simulink model "circuitExample"  (R2021b)
settings: Solver=VariableStepAuto  StartTime=0.0  StopTime=10.0  RelTol=1e-6
libraries: fl_lib x8, nesl_utility x1
settings Model: Creator=Rocksmithed  LastModifiedBy=Work

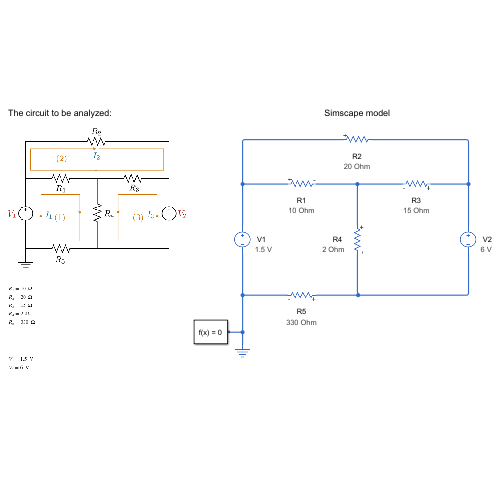
[thumbnail: Simulink's stored preview of the top-level diagram]
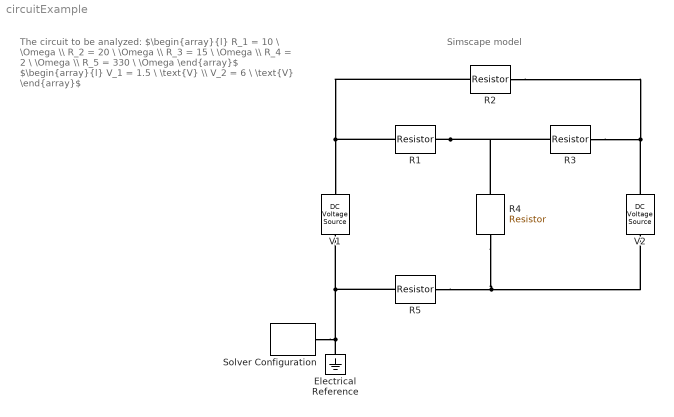
== system circuitExample ==
  note: Simscape model
  note: The circuit to be analyzed:
      |
      | $\begin{array}{l} R_1 = 10 \ \Omega \\ R_2 = 20 \ \Omega \\ R_3 = 15 \ \Omega \\ R_4 = 2 \ \Omega \\ R_5 = 330 \ \Omega \end{array}$
      |
      | $\begin{array}{l} V_1 = 1.5 \ \text{V} \\ V_2 = 6 \ \text{V} \end{array}$
  Electrical Reference : fl_lib/Electrical/Electrical Elements/Electrical Reference
  R1 : fl_lib/Electrical/Electrical Elements/Resistor  R=10 Ohm  i_specify=off  i_priority=None  i=0 A  i_nominal_specify=off  i_nominal_unit=A  i_nominal_value=1  v_specify=off  v_priority=None  v=0 V  v_nominal_specify=off  v_nominal_unit=V  v_nominal_value=1
      settings: AttributesFormatString=%<R> %<R_unit>
  R2 : fl_lib/Electrical/Electrical Elements/Resistor  R=20 Ohm  i_specify=off  i_priority=None  i=0 A  i_nominal_specify=off  i_nominal_unit=A  i_nominal_value=1  v_specify=off  v_priority=None  v=0 V  v_nominal_specify=off  v_nominal_unit=V  v_nominal_value=1
      settings: AttributesFormatString=%<R> %<R_unit>
  R3 : fl_lib/Electrical/Electrical Elements/Resistor  R=15 Ohm  i_specify=off  i_priority=None  i=0 A  i_nominal_specify=off  i_nominal_unit=A  i_nominal_value=1  v_specify=off  v_priority=None  v=0 V  v_nominal_specify=off  v_nominal_unit=V  v_nominal_value=1
      settings: AttributesFormatString=%<R> %<R_unit>
  R4 : fl_lib/Electrical/Electrical Elements/Resistor  R=2 Ohm  i_specify=off  i_priority=None  i=0 A  i_nominal_specify=off  i_nominal_unit=A  i_nominal_value=1  v_specify=off  v_priority=None  v=0 V  v_nominal_specify=off  v_nominal_unit=V  v_nominal_value=1
      settings: AttributesFormatString=%<R> %<R_unit>
  R5 : fl_lib/Electrical/Electrical Elements/Resistor  R=330 Ohm  i_specify=off  i_priority=None  i=0 A  i_nominal_specify=off  i_nominal_unit=A  i_nominal_value=1  v_specify=off  v_priority=None  v=0 V  v_nominal_specify=off  v_nominal_unit=V  v_nominal_value=1
      settings: AttributesFormatString=%<R> %<R_unit>
  Solver Configuration : nesl_utility/Solver Configuration  PhysicalDomain=network_engine_domain  SubClassName=solver  LeftPortType=input  RightPortType=generic  Tones=[]  Harmonics=[]  SimulateNoise=off  Profile=off  UseLocalSampling=off  EnableSwitchedLinearOptims=on  FrequencyDomain=off  UseCCode=off  RelTol=0.001  AbsTol=1e-06  MinStep=1e-09  ToWorkspace=off  RevertToSquareIcSolve=off  NumHomotopyIterations=100  PhasorMode=off  PhasorModeNumHarmonics=1  DoDC=off  ResidualTolerance=1e-09  UseLocalSolver=off  LocalSolverChoice=NE_BACKWARD_EULER_ADVANCER  LocalSolverSampleTime=0.001  DoFixedCost=off  MaxNonlinIter=3  MaxModeIter=2  ComputeImpulses=off  ImpulseIterations=2  LinearAlgebra=auto  EquationFormulation=NE_TIME_EF  DelaysMemoryBudget=1024  AutomaticFiltering=on  FilteringTimeConstant=0.001  PartitionStorageMethod=AS_NEEDED  PartitionMemoryBudget=1024  PartitionMethod=ROBUST
      settings: SourceProductBaseCode=PW,SS
  V1 : fl_lib/Electrical/Electrical Sources/DC Voltage Source  v0=1.5 V
      settings: AttributesFormatString=%<v0> %<v0_unit>
  V2 : fl_lib/Electrical/Electrical Sources/DC Voltage Source  v0=6 V
      settings: AttributesFormatString=%<v0> %<v0_unit>
  connections:
  R1/LConn1 -- R2/LConn1 -- V1/LConn1
  R1/RConn1 -- R3/RConn1 -- R4/LConn1
  R2/RConn1 -- R3/LConn1 -- V2/LConn1
  R4/RConn1 -- R5/LConn1 -- V2/RConn1
  Electrical Reference/LConn1 -- Solver Configuration/RConn1 -- R5/RConn1 -- V1/RConn1
